simulink subsystem "single_cell"  (R2021a)
settings: Solver=VariableStepAuto  StartTime=0.0  StopTime=10.0  RelTol=1e-3
libraries: fl_lib x5, nesl_utility x4, ee_lib x1
settings Model: Creator=Carlo Edoardo  LastModifiedBy=Carlo Edoardo

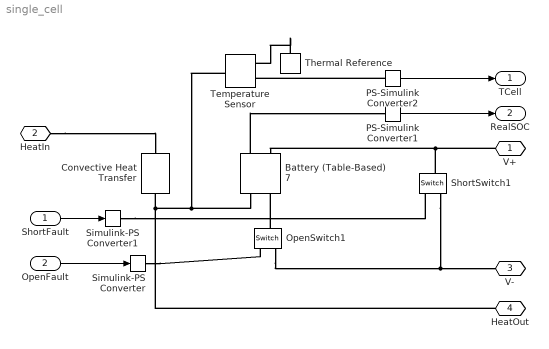
== system single_cell ==
  ShortFault : Inport
  OpenFault : Inport  Port=2
  Battery (Table-Based)7 : ee_lib/Sources/Battery (Table-Based)  Tag={'toolbox/physmod/elec/library/m/ee_lib_parts';'Sources/Battery__Table_Based_/A123/AMP20M1HD.xml'}  SOC_vec=[0.01 0.02 0.03 0.04 0.05 0.06 0.07 0.08 0.09 0.1 0.11 0.12 0.13 0.14 0.15 0.16 0.17 0.18 0.19 0.2 0.21 0.22 0.23 0.24 0.25 0.26 0.27 0.28 0.29 0.3 0.31 0.32 0.33 0.34 0.35 0.36 0.37 0.38 0.39 0.4 0.41 0.42 0.43 0.44 0.45 0.46 0.47 0.48 0.49 0.5 0.51 0.52 0.53 0.54 0.55 0.56 0.57 0.58 0.59 0.6 0.61 0.62 0.63 0.64 0.65 0.66 0.67 0.68 0.69 0.7 0.71 0.72 0.73 0.74 0.75 0.76 0.77 0.78 0.79 0.8 0.81 0.82 0.83 0.84 0.85 0.86 0.87 0.88 0.89 0.9 0.91 0.92 0.93 0.94 0.95 0.96 0.97 0.98 0.99 1]  T_dependence=ee.enum.temperature_dependence.yes  prm_dir=ee.enum.battery.prm_dir.noCurrentDirectionality  T_vec=[-10 0 10 25 35 45] degC  V0_mat=[2.02048467956871 2.02552449023345 2.00241395976794 2.65303897660795 2.01946900690675 2.01027487918888;2.04779238619957 2.07078499061078 2.08510164032757 2.73455624589417 2.59400684441827 2.63368825516668;2.07505500882737 2.11572219493149 2.16731902140654 2.80344516549462 2.69901543539581 2.8121655499412;2.10225818630398 2.16062213147566 2.23134769120249 2.86264890028114 2.79963633738328 2.88358256799339;2.12941122137965 2.20553359282369 2.29141771751294 2.91133273456944 2.90025721426303 2.95499956813595;2.156541005023 2.25040646018699 2.35096073589964 2.95146046787967 2.98369015639774 3.02641655036932;2.18367606614453 2.294749098711 2.40586898655962 2.98551519476444 3.01317154377941 3.05281487784124;2.2108321078396 2.33730664060215 2.4600933272137 3.01639186347584 3.04265292380958 3.07569862690579;2.23900676545081 2.38001405729144 2.51426094718943 3.03661530064054 3.07213429648844 3.09858237023656;2.26874057385119 2.42299251648117 2.56844448312329 3.05557903380075 3.09224038902396 3.1115993241461;2.29843391052372 2.46599091029475 2.62256559944252 3.07429344278984 3.10307831765322 3.12068440668465;2.32809013427346 2.50819084614007 2.66786053895406 3.08906455594511 3.11391624358426 3.12971593586611;2.35774593755925 2.54671248983025 2.71010724515821 3.09893170534327 3.11782408956293 3.13331743618893;2.38743256302521 2.58515598763761 2.75256052825076 3.10827161494006 3.12139575748141 3.136918935615;2.41711717370944 2.62356748428262 2.79534601117573 3.11817353363478 3.12496742451509 3.14052043414434;2.44617414251787 2.66199377409788 2.83810355336983 3.12853805169897 3.12853909066401 3.14412193177698;2.47490113758924 2.69827352673971 2.87544646360341 3.13602904737529 3.13211075592818 3.14772342851294;2.50362842838308 2.72743063564978 2.9103486532254 3.14237958250933 3.13568242030762 3.15132492435224;2.53235443586739 2.75656747444858 2.94516332887887 3.14776764345559 3.13925408380236 3.1549264192949;2.5610787022988 2.78563985754237 2.97792514507794 3.15244645705239 3.14282574641241 3.15852791334095;2.58979939734078 2.81467952754887 2.99139452296034 3.15712527064919 3.14639740813781 3.16212940649041;2.61749222516001 2.84027612484396 3.00489276327287 3.16123979887733 3.14996906897857 3.1657308987433;2.6384061317037 2.85749172776215 3.01839068088464 3.16498623188047 3.15354072893471 3.16928534893461;2.65931783314313 2.87470613098749 3.03180691985593 3.16873266488361 3.15711238800627 3.17281923730315;2.6802279296263 2.89192787101372 3.04516663256063 3.17147673469933 3.16068404619325 3.17635312479214;2.70114715503656 2.90915068936977 3.05859730772979 3.17370382586369 3.16425570349569 3.17988701140161;2.72112525437787 2.92637267894582 3.06512422104882 3.17612813890507 3.1678273599136 3.18342089713157;2.73466363338249 2.93797131395005 3.07147027491555 3.17855245194644 3.17139901544701 3.18695478198206;2.74818354277056 2.94941755810633 3.07782540168639 3.18097676498781 3.17497067009595 3.19048866595309;2.76164981161808 2.96084896827219 3.08418290085332 3.18327462462441 3.17766812517877 3.19402254904469;2.77511329525926 2.97227429025246 3.0905402962562 3.18554901437863 3.17982885815415 3.19755643125688;2.78857909694872 2.98369874846827 3.09689738603447 3.18782340413285 3.18198959059709 3.20099475363232;2.80204453896681 2.99109750499242 3.10323573691381 3.19009779388708 3.18415032250762 3.20288851688606;2.81550909850105 2.9964319812083 3.10955893632495 3.19207799320467 3.18631105388574 3.20478227967169;2.82897277630068 3.00181257824455 3.11228247869481 3.19386863504757 3.18847178473147 3.20667604198922;2.83947261373766 3.00716290217952 3.11448158268586 3.19565927689048 3.19063251504483 3.20856980383867;2.84611192000047 3.01245320885601 3.11670930669159 3.19744991873338 3.19279324482582 3.21046356522005;2.8527508171283 3.017752528873 3.11900915326186 3.19932802614273 3.19495397407446 3.21235732613336;2.85938930546812 3.0207113026139 3.1213061088066 3.20140875884178 3.19711470279077 3.21425108657863;2.86602738536648 3.02356810945713 ...(+6150 chars)] V  V0_vec=[2.65303897660795 2.73455624589417 2.80344516549462 2.86264890028114 2.91133273456944 2.95146046787967 2.98551519476444 3.01639186347584 3.03661530064054 3.05557903380075 3.07429344278984 3.08906455594511 3.09893170534327 3.10827161494006 3.11817353363478 3.12853805169897 3.13602904737529 3.14237958250933 3.14776764345559 3.15244645705239 3.15712527064919 3.16123979887733 3.16498623188047 3.16873266488361 3.17147673469933 3.17370382586369 3.17612813890507 3.17855245194644 3.18097676498781 3.18327462462441 3.18554901437863 3.18782340413285 3.19009779388708 3.19207799320467 3.19386863504757 3.19565927689048 3.19744991873338 3.19932802614273 3.20140875884178 3.20329846428421 3.20458294399616 3.20572972073489 3.20685938914037 3.20798905754585 3.20911872595133 3.21024839435682 3.2113780627623 3.21250773116778 3.21363739957326 3.21476706797874 3.21589673638422 3.21689328427519 3.21801321354037 3.21913314280554 3.22025272169618 3.22137150153786 3.22249597229506 3.2236244896631 3.22475300703114 3.22588152439919 3.22701004176723 3.22813855913527 3.22926707650332 3.23039559387136 3.23152411123941 3.23265262860745 3.23378114597549 3.23490880549975 3.23595318293068 3.23694933188764 3.23820579547914 3.23946225907064 3.24085615344745 3.24250847849207 3.24416080353669 3.24581312858131 3.24746545362594 3.24911777867056 3.25077010371518 3.2524224287598 3.25407475380442 3.25572707884905 3.25737940389367 3.25906640064108 3.26075478766727 3.26197307071463 3.2629039987276 3.26332953050402 3.26375506228044 3.26418059405687 3.26460612583329 3.26503165760971 3.26574042679347 3.26598762333395 3.26642291992706 3.26772852834402 3.26903413676098 3.27751094002651 3.2848395263804 3.30513945358125] V  R0_mat=[0.00106491718595769 0.00118733090981592 0.000475901485932642 0.000333306725149987 0.000815987550117719 0.000812269688087543;0.00108164289202854 0.00122615493026713 0.000754112991855717 0.00065822848128496 0.00104814285152977 0.0010641729179463;0.00109871383990162 0.00123207396062963 0.000973536296818726 0.00090219927789565 0.0010905805453475 0.00113629672055161;0.0011109767468834 0.00123788269635515 0.00114196673801776 0.00112492330446318 0.00113124590035651 0.00116516195401928;0.00111907300376166 0.00124601943167631 0.00127797700112948 0.00129677992117799 0.00117191181029675 0.00119402758332599;0.00112522551953292 0.00126226743857129 0.00136989648804215 0.00141844628190335 0.00120563307932694 0.00122289360846161;0.00113200127210202 0.00126402231459423 0.00142880013594437 0.00150118311426028 0.00121755421834844 0.00123356908083094;0.00114114494599905 0.00125994922803471 0.00143552713314253 0.00156760818891277 0.00122947551985284 0.00124282453555034;0.00115263378066748 0.00126215372635823 0.00144200280404935 0.00159930387330856 0.00124139698383596 0.00125208011699765;0.00116485196460463 0.00127767161018923 0.00145116268236509 0.00162412719543218 0.00124953019639963 0.0012573488115951;0.00117614142055791 0.00130182742270516 0.00146990247761868 0.00164958981030225 0.00125391836299715 0.00126102876046515;0.00118566775080578 0.00132756996177559 0.00146648644380373 0.00166733382622861 0.00125830658923075 0.00126468712009524;0.00119478622254968 0.00134604950823589 0.00145693025409017 0.00165632701229496 0.00125989447143005 0.00126615129451334;0.00120526654851145 0.00135803525806723 0.00145636607855883 0.00164194045604481 0.00126134652690013 0.00126761548875141;0.00121563816945444 0.00136734174721288 0.00147310646561793 0.00164023513072252 0.00126279860192591 0.001269079702809;0.00122558784624188 0.00137834967586499 0.00149943126737675 0.00166007639811452 0.00126425069650694 0.00127054393668553;0.00123592755710294 0.00139140066231826 0.00152303079157175 0.00167340129602339 0.0012657028106427 0.00127200819038055;0.00124641069998859 0.0014023366360332 0.00153577814235498 0.00168050436882428 0.00126715494433267 0.00127347246389355;0.00125686160761269 0.00141277808909305 0.00154125890410489 0.00168143773529334 0.00126860709757642 0.00127493675722402;0.00126722920089371 0.00142133550347284 0.00154543792168517 0.00167782464439403 0.00127005927037337 0.00127640107037144;0.00127752492966828 0.00142754428848147 0.00154439925657168 0.0016742115534947 0.0012715114627231 0.00127786540333531;0.00128732460357676 0.00143453799871213 0.00154658499182436 0.00167204534815603 0.00127296367462507 0.00127932975611514;0.00129378668080401 0.00143721679045437 0.00154875227798245 0.00167082297672762 0.00127441590607878 0.00128077511838248;0.00130019584417818 0.0014398308542752 0.00154912946249455 0.00166960060529919 0.00127586815708375 0.00128221219103687;0.00130654853180782 0.0014433285393301 0.00154583302343157 0.0016627165979173 0.00127732042763948 0.00128364928313102;0.00131332542787091 0.00144701431023556 0.00154565339925959 0.00165283682176085 0.00127877271774547 0.00128508639466439;0.00132091956369151 0.00145067611662764 0.00154214182084189 0.00164740718026511 0.00128022502740126 0.00128652352563652;0.00132740526853119 0.00145150880812309 0.00153852059904326 0.00164197753876937 0.0012816773566063 0.00128796067604689;0.00133238713298699 0.00145231822127064 0.00153592694539016 0.00163654789727363 0.0012831297053601 0.00128939784589505;0.00133296918209426 0.00145318305444644 0.00153361631405066 0.00163144249527728 0.00128422877336262 0.00129083503518046;0.00133351371086521 0.00145404956550509 0.00153131353131826 0.00162639727246654 0.00128511094297309 0.00129227224390263;0.00133436260205017 0.00145488568212758 0.00152899612357707 0.00162135204965579 0.0012859931243514 0.00129367085224213;0.00133521829148733 0.00145427389454777 0.00152677756437621 0.00161630682684504 0.00128687531749717 0.00129444524729978;0.00133602264918931 0.00145456100370279 ...(+7957 chars)] Ohm  R0_vec=[0.000333306725149987 0.00065822848128496 0.00090219927789565 0.00112492330446318 0.00129677992117799 0.00141844628190335 0.00150118311426028 0.00156760818891277 0.00159930387330856 0.00162412719543218 0.00164958981030225 0.00166733382622861 0.00165632701229496 0.00164194045604481 0.00164023513072252 0.00166007639811452 0.00167340129602339 0.00168050436882428 0.00168143773529334 0.00167782464439403 0.0016742115534947 0.00167204534815603 0.00167082297672762 0.00166960060529919 0.0016627165979173 0.00165283682176085 0.00164740718026511 0.00164197753876937 0.00163654789727363 0.00163144249527728 0.00162639727246654 0.00162135204965579 0.00161630682684504 0.00160965663711322 0.0016019723094944 0.00159428798187562 0.0015866036542568 0.00158089290865004 0.00157975422086216 0.00157739099937799 0.00157114812577538 0.00156525833671951 0.00155941241518479 0.00155356649365008 0.00154772057211534 0.00154187465058062 0.00153602872904589 0.00153018280751117 0.00152433688597645 0.00151849096444173 0.001512645042907 0.00150619130440395 0.00150316935092012 0.0015001473974363 0.00149712319796183 0.00149409387637865 0.00149104996270438 0.00148799567310486 0.00148494138350538 0.00148188709390585 0.00147883280430635 0.00147577851470684 0.00147272422510734 0.00146966993550782 0.00146661564590832 0.0014635613563088 0.0014605070667093 0.00145744809711094 0.00145420114928265 0.00145292480649112 0.00145752222981219 0.00146211965313325 0.00146759804302683 0.00147473303976536 0.00148186803650389 0.00148900303324241 0.00149613802998095 0.00150327302671948 0.001510408023458 0.00151754302019654 0.00152467801693506 0.0015318130136736 0.00153894801041212 0.00154599410534863 0.00155303663546773 0.00155706567854303 0.00155704809705804 0.0015468366366642 0.00153662517627038 0.00152641371587654 0.00151620225548271 0.00150599079508888 0.00149759495910105 0.00146548197254331 0.00143133809444856 0.00139496264757467 0.0013585872007008 0.00136444083816036 0.00129932822636862 0.00127867578328036] Ohm  R0_dis_mat=[0.03 0.015 0.002;0.04 0.017 0.008;0.039 0.012 0.006;0.027 0.013 0.021] % Parameter not set Ohm  R0_dis_vec=[0.015 0.017 0.012 0.013] % Parameter not set Ohm  R0_ch_mat=[0.03 0.015 0.002;0.04 0.017 0.008;0.039 0.012 0.006;0.027 0.013 0.021] % Parameter not set Ohm  R0_ch_vec=[0.015 0.017 0.012 0.013] % Parameter not set Ohm  AH_vec=[15.8082703950129 17.433405393 18.3937700370255 18.6255821924799 0.019486598769882 0.0195859468365053] hr*A  AH=18.6255821924799 hr*A  prm_leak=ee.enum.battery.prm_leak.disabled  Rleak_vec=[8000 7000 6000] % Parameter not set Ohm  Rleak=7000 % Parameter not set Ohm  extrapolation_option=ee.enum.extrapolation.nearest  prm_dyn=ee.enum.battery.prm_dyn.off  R1_mat=[0.089 0.076 0.01;0.042 0.022 0.099;0.019 0.007 0.002;0.051 0.043 0.029] % Parameter not set Ohm  R1_vec=[0.076 0.022 0.007 0.043] % Parameter not set Ohm  tau1_mat=[44 148 235;93 110 1000;19 27 133;0.5 22 3] % Parameter not set s  tau1_vec=[148 110 27 22] % Parameter not set s  R2_mat=[0.014 0.382 0.407;0.028 0.006 0.007;0.014 0.007 0.006;0.333 0.956 0.912] % Parameter not set Ohm  R2_vec=[0.382 0.006 0.007 0.956] % Parameter not set Ohm  tau2_mat=[1 44 5644;11 24 506;2 14 330;3310 13419 30216] % Parameter not set s  tau2_vec=[44 24 14 13419] % Parameter not set s  R3_mat=[0.014 0.382 0.407;0.028 0.006 0.007;0.014 0.007 0.006;0.333 0.956 0.912] % Parameter not set Ohm  R3_vec=[0.382 0.006 0.007 0.956] % Parameter not set Ohm  tau3_mat=[1 44 5644;11 24 506;2 14 330;3310 13419 30216] % Parameter not set s  tau3_vec=[44 24 14 13419] % Parameter not set s  R4_mat=[0.014 0.382 0.407;0.028 0.006 0.007;0.014 0.007 0.006;0.333 0.956 0.912] % Parameter not set Ohm  R4_vec=[0.382 0.006 0.007 0.956] % Parameter not set Ohm  tau4_mat=[1 44 5644;11 24 506;2 14 330;3310 13419 30216] % Parameter not set s  tau4_vec=[44 24 14 13419] % Parameter not set s  R5_mat=[0.014 0.382 0.407;0.028 0.006 0.007;0.014 0.007 0.006;0.333 0.956 0.912] % Parameter not set Ohm  R5_vec=[0.382 0.006 0.007 0.956] % Parameter not set Ohm  tau5_mat=[1 44 5644;11 24 506;2 14 330;3310 13419 30216] % Parameter not set s  tau5_vec=[44 24 14 13419] % Parameter not set s  prm_fade=ee.enum.battery.prm_fade.tableN  N0=100 % Parameter not set  dV0=0 % Parameter not set  dR0=0 % Parameter not set  dAH=0 % Parameter not set  dRleak=0 % Parameter not set  dR1=0 % Parameter not set  dR2=0 % Parameter not set  dR3=0 % Parameter not set  dR4=0 % Parameter not set  dR5=0 % Parameter not set  N0vec=[1 66 131 196 261 326 391 456 521 586 651 716 781 846 911 976 1041 1106 1171 1236 1301 1366 1431 1496 1561 1626 1691 1756 1821 1886 1951 2016 2081 2146 2211 2276 2341 2406 2471 2536 2601 2666 2731 2796 2861 2926 2991 3056 3121 3186 3251 3316 3381 3446 3511 3576 3641 3706 3771 3836 3901 3966 4031 4096 4161 4226 4291 4356 4421 4486 4551 4616 4681 4746 4811 4876 4941 5006 5071 5136 5201 5266 5331 5396 5461 5526 5591 5656 5721 5786 5851 5916 5981 6046 6111 6176 6241 6306 6371 6436]  Tfadevec=[298.15 323.15] % Parameter not set K  dV0vec=[0 -0.195792036901586 -0.391584073803145 -0.576964570915662 -0.656113365994186 -0.711473922188788 -0.766834478383404 -0.82219503457802 -0.884077998062453 -0.947586707636299 -1.0109664570589 -1.0743462064815 -1.09938048339923 -1.1091423159815 -1.11890414856378 -1.12866598114604 -1.13856480277705 -1.14852228326816 -1.15847976375928 -1.1684372442504 -1.17373470118599 -1.17705457663823 -1.18037445209049 -1.18369432754273 -1.1859598437997 -1.18784513704483 -1.18968175971891 -1.19143518795745 -1.19530835027982 -1.20033583124303 -1.20536331220624 -1.21039079316945 -1.21465083390349 -1.21766923954839 -1.22068764519332 -1.22370605083822 -1.22679421316894 -1.23012729929626 -1.23346038542359 -1.23679347155092 -1.24012655767824 -1.24345964380556 -1.24679272993288 -1.25012581606021 -1.25345890218753 -1.25679198831485 -1.26012507444217 -1.26345816056949 -1.26669937212443 -1.26981111846062 -1.2729228647968 -1.27603461113299 -1.28065977277097 -1.28746728279512 -1.29427479281927 -1.30108230284341 -1.30846137009002 -1.31737019434028 -1.32627901859052 -1.33518784284078 -1.3446964360184 -1.35723928501926 -1.3697821340201 -1.38232498302095 -1.3948671026925 -1.40739962345903 -1.41993214422557 -1.43262513753545 -1.44535603285615 -1.45783210812411 -1.47030818339207 -1.48278425866 -1.49526033392796 -1.50773640919596 -1.52021248446395 -1.5326350134729 -1.54497285638699 -1.55731069930105 -1.56964854221509 -1.58198638512916 -1.5943242280432 -1.60666207095727 -1.61899991387136 -1.63133775678545 -1.64364794564584 -1.65592289399208 -1.66819784233834 -1.68047279068458 -1.69274773903082 -1.70502268737707 -1.71729763572331 -1.72957258406955 -1.74215202312793 -1.75493538987971 -1.76771875663151 -1.78050212338331 -1.79328549013512 -1.80606885688686 -1.81885222363863 -1.83163559039039]  dR0vec=[0;0;0;0;0;0;0;0;0;0;0;0;0;0;0;0;0;0;0;0;0;0;0;0;0;0;0;0;0;0;0;0;0;0;0;0;0;0;0;0;0;0;0;0;0;0;0;0;0;0;0;0;0;0;0;0;0;0;0;0;0;0;0;0;0;0;0;0;0;0;0;0;0;0;0;0;0;0;0;0;0;0;0;0;0;0;0;0;0;0;0;0;0;0;0;0;0;0;0;0] % Parameter not set  dAHvec=[0 -0.318779461353655 -0.63755892270731 -0.939386800644478 -1.18905890603464 -1.43873101142481 -1.68840311681495 -1.93807522220512 -2.18774732759526 -2.43537032306114 -2.68249049774603 -2.9296106724309 -3.17673084711578 -3.42385102180065 -3.67097119648554 -3.91809137117043 -4.16867941496321 -4.42075240409153 -4.67282539321987 -4.92489838234821 -5.17697137147655 -5.42904436060487 -5.68111734973321 -5.93319033886155 -6.18526332798989 -6.43733631711823 -6.68290181126916 -6.91734379978052 -7.15178578829185 -7.38622777680321 -7.62066976531457 -7.85511175382591 -8.08955374233725 -8.32399573084861 -8.55843771935995 -8.7928797078713 -9.03273975414459 -9.29162322823482 -9.55050670232507 -9.80939017641532 -10.0682736505056 -10.3271571245958 -10.5860405986861 -10.8449240727763 -11.1038075468666 -11.3626910209568 -11.6215744950471 -11.8804579691373 -12.1322054714672 -12.3738973063685 -12.6155891412699 -12.8572809761712 -13.0989728110726 -13.3406646459739 -13.5823564808753 -13.8240483157766 -14.065740150678 -14.3074319855794 -14.5491238204807 -14.7908156553821 -15.0351972165451 -15.2807325378302 -15.5262678591153 -15.7718031804005 -16.0173385016855 -16.2628738229706 -16.5084091442557 -16.7570884202344 -17.0066468756258 -17.2562053310172 -17.5057637864085 -17.7553222417999 -18.0048806971913 -18.2544391525826 -18.503997607974 -18.7524849795981 -18.9992783785124 -19.2460717774268 -19.4928651763412 -19.7396585752556 -19.9864519741699 -20.2332453730843 -20.4800387719986 -20.726832170913 -20.9730724068515 -21.2186077281366 -21.4641430494217 -21.7096783707068 -21.9552136919919 -22.200749013277 -22.4462843345621 -22.6918196558472 -22.9434456931763 -23.1991508883401 -23.4548560835039 -23.7105612786676 -23.9662664738314 -24.2219716689951 -24.4776768641589 -24.7333820593227]  dRleakvec=[0 0 0] % Parameter not set  dR1vec=[0 0 0] % Parameter not set  dR2vec=[0 0 0] % Parameter not set  dR3vec=[0 0 0] % Parameter not set  dR4vec=[0 0 0] % Parameter not set  dR5vec=[0 0 0] % Parameter not set  dV0mat=[0 0;0 0;0 0] % Parameter not set  dR0mat=[0 0;0 0;0 0] % Parameter not set  dAHmat=[0 0;0 0;0 0] % Parameter not set  dRleakmat=[0 0;0 0;0 0] % Parameter not set  dR1mat=[0 0;0 0;0 0] % Parameter not set  dR2mat=[0 0;0 0;0 0] % Parameter not set  dR3mat=[0 0;0 0;0 0] % Parameter not set  dR4mat=[0 0;0 0;0 0] % Parameter not set  dR5mat=[0 0;0 0;0 0] % Parameter not set  prm_age=ee.enum.battery.prm_age.disabled  prm_age_OCV=ee.enum.battery.prm_age_OCV.SOC  OCV_age=0.9 % Parameter not set  SOC_age=0.6 % Parameter not set  storage_dt_age_vec=0 % Parameter not set d  storage_T_age_vec=273 % Parameter not set K  OCV_scaling_age=2213400 % Parameter not set  OCV_offset_age=1632000 % Parameter not set  temp_exp_age=0.515833569 % Parameter not set V  t_exp_age=0.75 % Parameter not set  T_age_vec=[273.15 298.15 323.15] % Parameter not set K  dt_age_vec=[90 180 270 360] % Parameter not set d  dR0_age_vec=[0 0 0] % Parameter not set  t_meas_dR0_age=100 % Parameter not set d  dR0_age_mat=[0 0 0;0 0 0;0 0 0;0 0 0] % Parameter not set  temperature=298.15 K  i_specify=off  i_priority=None  i=0 A  i_nominal_specify=off  i_nominal_unit=A  i_nominal_value=1  v_specify=off  v_priority=None  v=0 V  v_nominal_specify=off  v_nominal_unit=V  v_nominal_value=1  stateOfCharge_specify=on  stateOfCharge_priority=High  stateOfCharge=1  stateOfCharge_nominal_specify=off  stateOfCharge_nominal_unit=1  stateOfCharge_nominal_value=1  num_cycles_specify=off  num_cycles_priority=High  num_cycles=0  num_cycles_nominal_specify=off  num_cycles_nominal_unit=1  num_cycles_nominal_value=1  thermal_mass=30000 % Parameter not set J/K  temperature_specify=on  temperature_priority=High  temperature_nominal_specify=off  temperature_nominal_unit=K  temperature_nominal_value=1
      settings: AttributesFormatString=A123:AMP20M1HD  SourceProductBaseCode=PS  InternalSimscapePortConfiguration="{\"Bottom\":[],\"Left\":[{\"id\":\"p\",\"label\":\"+\",\"type\":\"foundation.electrical.electrical\"},{\"id\":\"soc\",\"label\":\"SOC\",\"type\":\"output\"}],\"Right\":[{\"id\":\"n\",\"label\":\"-\",\"type\":\"foundation.electrical.electrical\"},{\"id\":\"H\",\"label\":\"H\",\"type\":\"foundation.thermal.thermal\"}],\"Top\":[]}"
  Convective Heat Transfer : fl_lib/Thermal/Thermal Elements/Convective Heat Transfer  area=1e-4 m^2  heat_tr_coeff=20 W/(m^2 * K)  T_specify=off  T_priority=None  T=0 K  T_nominal_specify=off  T_nominal_unit=K  T_nominal_value=1  Q_specify=off  Q_priority=None  Q=0 W  Q_nominal_specify=off  Q_nominal_unit=W  Q_nominal_value=1
  OpenSwitch1 : fl_lib/Electrical/Electrical Elements/Switch  R_closed=1e-12 Ohm  G_open=1e-10 1/Ohm  Threshold=0  i_specify=off  i_priority=None  i=0 A  i_nominal_specify=off  i_nominal_unit=A  i_nominal_value=1  v_specify=off  v_priority=None  v=0 V  v_nominal_specify=off  v_nominal_unit=V  v_nominal_value=1
  PS-Simulink Converter1 : nesl_utility/PS-Simulink Converter  PhysicalDomain=network_engine_domain  SubClassName=ps_output  LeftPortType=input  RightPortType=output  PseudoPeriodic=off  Frequencies=[]  Unit=inherit  AffineConversion=off
      settings: SourceProductBaseCode=PW,SS
  PS-Simulink Converter2 : nesl_utility/PS-Simulink Converter  PhysicalDomain=network_engine_domain  SubClassName=ps_output  LeftPortType=input  RightPortType=output  PseudoPeriodic=off  Frequencies=[]  Unit=inherit  AffineConversion=off
      settings: SourceProductBaseCode=PW,SS
  ShortSwitch1 : fl_lib/Electrical/Electrical Elements/Switch  R_closed=1e-10 Ohm  G_open=1e-10 1/Ohm  Threshold=0.5  i_specify=off  i_priority=None  i=0 A  i_nominal_specify=off  i_nominal_unit=A  i_nominal_value=1  v_specify=off  v_priority=None  v=0 V  v_nominal_specify=off  v_nominal_unit=V  v_nominal_value=1
  Simulink-PS Converter : nesl_utility/Simulink-PS Converter  PhysicalDomain=network_engine_domain  SubClassName=ps_input  LeftPortType=input  RightPortType=output  PseudoPeriodic=off  Frequencies=[]  NoiseDistribution=none  NoiseParameters=[]  Unit=1  AffineConversion=off  FilteringAndDerivatives=provide  SimscapeFilterOrder=1  InputFilterTimeConstant=0.001  UdotUserProvided=0
      settings: SourceProductBaseCode=PW,SS
  Simulink-PS Converter1 : nesl_utility/Simulink-PS Converter  PhysicalDomain=network_engine_domain  SubClassName=ps_input  LeftPortType=input  RightPortType=output  PseudoPeriodic=off  Frequencies=[]  NoiseDistribution=none  NoiseParameters=[]  Unit=1  AffineConversion=off  FilteringAndDerivatives=provide  SimscapeFilterOrder=1  InputFilterTimeConstant=0.001  UdotUserProvided=0
      settings: SourceProductBaseCode=PW,SS
  Temperature Sensor : fl_lib/Thermal/Thermal Sensors/Temperature Sensor
  Thermal Reference : fl_lib/Thermal/Thermal Elements/Thermal Reference
  V+ : PMIOPort  Side=Right
  HeatIn : PMIOPort  Port=2  Side=Left
  V- : PMIOPort  Port=3  Side=Right
  HeatOut : PMIOPort  Port=4  Side=Left
  TCell : Outport
  RealSOC : Outport  Port=2
  wires:
  ShortFault/1 -> Simulink-PS Converter1/1
  OpenFault/1 -> Simulink-PS Converter/1
  PS-Simulink Converter2/1 -> TCell/1
  PS-Simulink Converter1/1 -> RealSOC/1
  connections:
  Battery (Table-Based)7/RConn2 -- Convective Heat Transfer/RConn1 -- HeatOut/RConn1 -- Temperature Sensor/LConn1
  OpenSwitch1/RConn2 -- V-/RConn1 -- ShortSwitch1/RConn2
  V+/RConn1 -- ShortSwitch1/LConn1 -- Battery (Table-Based)7/LConn1
  Simulink-PS Converter1/RConn1 -- ShortSwitch1/RConn1
  Battery (Table-Based)7/LConn2 -- PS-Simulink Converter1/LConn1
  Thermal Reference/LConn1 -- Temperature Sensor/RConn1
  PS-Simulink Converter2/LConn1 -- Temperature Sensor/RConn2
  Simulink-PS Converter/RConn1 -- OpenSwitch1/RConn1
  OpenSwitch1/LConn1 -- Battery (Table-Based)7/RConn1
  HeatIn/RConn1 -- Convective Heat Transfer/LConn1
